simulink library "mvt_blocks"  (Simulink 3.00)
values from neighbouring files (symbols this model uses):
  stack = struct('general',[],'evaluation',[],'simulation',[],'temp',[])    [gohome.m]
libraries: mvt_blocks x1
(part 1 of 2)

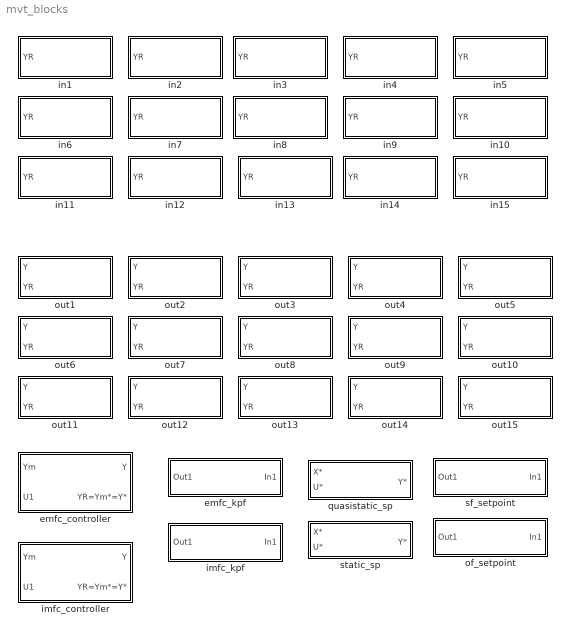
== system mvt_blocks ==
  emfc_controller : Subsystem  Orientation=left
      mask Display: disp('CONTROLLER')
  emfc_kpf : Subsystem  Orientation=left
      mask Display: disp('Kpf')
  imfc_controller : Subsystem  Orientation=left
      mask Display: disp('CONTROLLER')
  imfc_kpf : Subsystem  Orientation=left
      mask Display: disp('Kpf')
  in1 : Subsystem  Orientation=left
      mask Display: disp('COMMANDS')
  in10 : Subsystem  Orientation=left
      mask Display: disp('COMMANDS')
  in11 : Subsystem  Orientation=left
      mask Display: disp('COMMANDS')
  in12 : Subsystem  Orientation=left
      mask Display: disp('COMMANDS')
  in13 : Subsystem  Orientation=left
      mask Display: disp('COMMANDS')
  in14 : Subsystem  Orientation=left
      mask Display: disp('COMMANDS')
  in15 : Subsystem  Orientation=left
      mask Display: disp('COMMANDS')
  in2 : Subsystem  Orientation=left
      mask Display: disp('COMMANDS')
  in3 : Subsystem  Orientation=left
      mask Display: disp('COMMANDS')
  in4 : Subsystem  Orientation=left
      mask Display: disp('COMMANDS')
  in5 : Subsystem  Orientation=left
      mask Display: disp('COMMANDS')
  in6 : Subsystem  Orientation=left
      mask Display: disp('COMMANDS')
  in7 : Subsystem  Orientation=left
      mask Display: disp('COMMANDS')
  in8 : Subsystem  Orientation=left
      mask Display: disp('COMMANDS')
  in9 : Subsystem  Orientation=left
      mask Display: disp('COMMANDS')
  of_setpoint : Subsystem  Orientation=left
      mask Display: disp('Kpf')
  out1 : Subsystem
      mask Display: disp('OUTPUTS')
  out10 : Subsystem
      mask Display: disp('OUTPUTS')
  out11 : Subsystem
      mask Display: disp('OUTPUTS')
  out12 : Subsystem
      mask Display: disp('OUTPUTS')
  out13 : Subsystem
      mask Display: disp('OUTPUTS')
  out14 : Subsystem
      mask Display: disp('OUTPUTS')
  out15 : Subsystem
      mask Display: disp('OUTPUTS')
  out2 : Subsystem
      mask Display: disp('OUTPUTS')
  out3 : Subsystem
      mask Display: disp('OUTPUTS')
  out4 : Subsystem
      mask Display: disp('OUTPUTS')
  out5 : Subsystem
      mask Display: disp('OUTPUTS')
  out6 : Subsystem
      mask Display: disp('OUTPUTS')
  out7 : Subsystem
      mask Display: disp('OUTPUTS')
  out8 : Subsystem
      mask Display: disp('OUTPUTS')
  out9 : Subsystem
      mask Display: disp('OUTPUTS')
  quasistatic_sp : Subsystem  Orientation=left
      mask Display: disp('quasi-static\n SET POINT')
  sf_setpoint : Subsystem  Orientation=left
      mask Display: disp('Kpf')
  static_sp : Subsystem  Orientation=left
      mask Display: disp('static\n SET POINT')

== system mvt_blocks/emfc_controller ==
  Y : Inport  Orientation=left  Port=1  PortWidth=-1  SampleTime=-1  DataType=auto
      settings: SignalType=auto
  YR=Ym*=Y* : Inport  Orientation=left  Port=2  PortWidth=-1  SampleTime=-1  DataType=auto
      settings: SignalType=auto
  CONTROLLER : StateSpace  Orientation=left  A=stack.simulation.Ak  B=stack.simulation.Bk  C=stack.simulation.Ck  D=stack.simulation.Dk  X0=0
  MODEL : StateSpace  Orientation=left  A=stack.simulation.Am  B=stack.simulation.Bm  C=eye(size(stack.simulation.Am))  D=zeros(size(stack.simulation.Am,1),size(stack.simulation.Bm,2))  X0=0
  Matrix Gain : Subsystem  Orientation=left  mask(Matrix Gain){K=stack.simulation.Kff}
      mask prompts: K "Gain matrix:"
      mask help: Matrix Gain.
      mask Help: Multiplies input vector by entered matrix to produce output vector (y=Au).
      mask Display: disp('Kff')
  Matrix Gain1 : Subsystem  Orientation=left  mask(Matrix Gain){K=stack.simulation.Cm}
      mask prompts: K "Gain matrix:"
      mask help: Matrix Gain.
      mask Help: Multiplies input vector by entered matrix to produce output vector (y=Au).
      mask Display: disp('Cm')
  Sum : Sum  Orientation=left  Inputs=++|  SaturateOnIntegerOverflow=on
  Ym : Outport  Orientation=left  Port=1
  U1 : Outport  Orientation=left  Port=2
  wires:
  YR=Ym*=Y*/1 -> MODEL/1
  Y/1 -> CONTROLLER/1
  Matrix Gain/1(Out1) -> Sum/2
  Sum/1 -> U1/1
  CONTROLLER/1 -> Sum/1
  MODEL/1 -> Matrix Gain/1(In1), Matrix Gain1/1(In1)
  Matrix Gain1/1(Out1) -> Ym/1

== system mvt_blocks/emfc_kpf ==
  note: U*
  note: X*
  In1 : Inport  Orientation=left  Port=1  PortWidth=-1  SampleTime=-1  DataType=auto
      settings: SignalType=auto
  Matrix Gain : Subsystem  Orientation=left  mask(Matrix Gain){K=stack.simulation.Kfb}
      mask prompts: K "Gain matrix:"
      mask help: Matrix Gain.
      mask Help: Multiplies input vector by entered matrix to produce output vector (y=Au).
      mask Display: disp('Kfb')
  Matrix Gain1 : Subsystem  Orientation=left  mask(Matrix Gain){K=stack.simulation.Kpf0}
      mask prompts: K "Gain matrix:"
      mask help: Matrix Gain.
      mask Help: Multiplies input vector by entered matrix to produce output vector (y=Au).
      mask Display: disp('Kpf_0')
  Sum : Sum  Orientation=left  Inputs=++-  SaturateOnIntegerOverflow=on
  setpoint : Subsystem  Orientation=left
      mask Display: disp('SET POINT')
  Out1 : Outport  Orientation=left  Port=1
  wires:
  setpoint/1(X*) -> Matrix Gain/1(In1)
  Matrix Gain/1(Out1) -> Sum/1
  setpoint/2(U*) -> Sum/2
  Matrix Gain1/1(Out1) -> Sum/3
  In1/1 -> setpoint/1(Y*), Matrix Gain1/1(In1)
  Sum/1 -> Out1/1

== system mvt_blocks/imfc_controller ==
  Y : Inport  Orientation=left  Port=1  PortWidth=-1  SampleTime=-1  DataType=auto
      settings: SignalType=auto
  YR=Ym*=Y* : Inport  Orientation=left  Port=2  PortWidth=-1  SampleTime=-1  DataType=auto
      settings: SignalType=auto
  CONTROLLER : StateSpace  Orientation=left  A=stack.simulation.Ak  B=stack.simulation.Bk  C=stack.simulation.Ck  D=stack.simulation.Dk  X0=0
  MODEL : StateSpace  Orientation=left  A=stack.simulation.Am  B=stack.simulation.Bm  C=stack.simulation.Cm  D=stack.simulation.Dm  X0=0
  Ym : Outport  Orientation=left  Port=1
  U1 : Outport  Orientation=left  Port=2
  wires:
  Y/1 -> CONTROLLER/1
  YR=Ym*=Y*/1 -> MODEL/1
  MODEL/1 -> Ym/1
  CONTROLLER/1 -> U1/1

== system mvt_blocks/imfc_kpf ==
  note: X*
  note: U*
  In1 : Inport  Orientation=left  Port=1  PortWidth=-1  SampleTime=-1  DataType=auto
      settings: SignalType=auto
  Matrix Gain : Subsystem  Orientation=left  mask(Matrix Gain){K=stack.simulation.Kfb}
      mask prompts: K "Gain matrix:"
      mask help: Matrix Gain.
      mask Help: Multiplies input vector by entered matrix to produce output vector (y=Au).
      mask Display: disp('Kfb')
  Sum : Sum  Orientation=left  Inputs=|++  SaturateOnIntegerOverflow=on
  setpoint : Subsystem  Orientation=left
      mask Display: disp('SET POINT')
  Out1 : Outport  Orientation=left  Port=1
  wires:
  Sum/1 -> Out1/1
  setpoint/2(U*) -> Sum/2
  Matrix Gain/1(Out1) -> Sum/1
  setpoint/1(X*) -> Matrix Gain/1(In1)
  In1/1 -> setpoint/1(Y*)

== system mvt_blocks/in1 ==
  note: YR1
  Gen 1 : SignalGenerator  Orientation=left  WaveForm=sine  Amplitude=0.000000  Frequency=1  Units=rad/sec
  Step 1 : Step  Orientation=left  Time=0  Before=0  After=1  SampleTime=0
  Sum : Sum  Orientation=left  Inputs=|++  SaturateOnIntegerOverflow=on
  YR : Outport  Orientation=left  Port=1
  wires:
  Step 1/1 -> Sum/2
  Gen 1/1 -> Sum/1
  Sum/1 -> YR/1

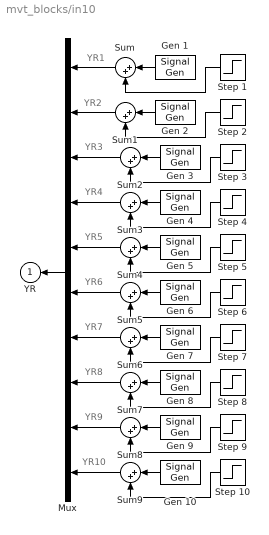
== system mvt_blocks/in10 ==
  note: YR1
  note: YR2
  note: YR3
  note: YR4
  note: YR5
  note: YR6
  note: YR7
  note: YR8
  note: YR9
  note: YR10
  Gen {1..10} (10 alike) : SignalGenerator  Orientation=left  WaveForm=sine  Amplitude=0.000000  Frequency=1  Units=rad/sec
  Mux : Mux  Orientation=left  Inputs=10
  Step {1..10} (10 alike) : Step  Orientation=left  Time=0  Before=0  After=1  SampleTime=0
  Sum{,1..9} (10 alike) : Sum  Orientation=left  Inputs=|++  SaturateOnIntegerOverflow=on
  YR : Outport  Orientation=left  Port=1
  wires:
  Sum/1 -> Mux/1
  Sum1/1 -> Mux/2
  Gen 1/1 -> Sum/1
  Mux/1 -> YR/1
  Sum3/1 -> Mux/4
  Sum4/1 -> Mux/5
  Step 1/1 -> Sum/2
  Gen 2/1 -> Sum1/1
  Step 2/1 -> Sum1/2
  Sum2/1 -> Mux/3
  Gen 3/1 -> Sum2/1
  Step 3/1 -> Sum2/2
  Gen 4/1 -> Sum3/1
  Step 4/1 -> Sum3/2
  Gen 5/1 -> Sum4/1
  Step 5/1 -> Sum4/2
  Sum5/1 -> Mux/6
  Gen 6/1 -> Sum5/1
  Step 6/1 -> Sum5/2
  Sum6/1 -> Mux/7
  Gen 7/1 -> Sum6/1
  Step 7/1 -> Sum6/2
  Sum7/1 -> Mux/8
  Gen 8/1 -> Sum7/1
  Step 8/1 -> Sum7/2
  Sum8/1 -> Mux/9
  Gen 9/1 -> Sum8/1
  Step 9/1 -> Sum8/2
  Sum9/1 -> Mux/10
  Gen 10/1 -> Sum9/1
  Step 10/1 -> Sum9/2

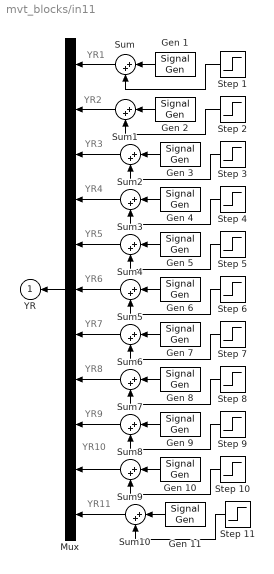
== system mvt_blocks/in11 ==
  note: YR1
  note: YR2
  note: YR3
  note: YR4
  note: YR5
  note: YR6
  note: YR7
  note: YR8
  note: YR9
  note: YR10
  note: YR11
  Gen {1..11} (11 alike) : SignalGenerator  Orientation=left  WaveForm=sine  Amplitude=0.000000  Frequency=1  Units=rad/sec
  Mux : Mux  Orientation=left  Inputs=11
  Step {1..11} (11 alike) : Step  Orientation=left  Time=0  Before=0  After=1  SampleTime=0
  Sum{,1..10} (11 alike) : Sum  Orientation=left  Inputs=|++  SaturateOnIntegerOverflow=on
  YR : Outport  Orientation=left  Port=1
  wires:
  Sum/1 -> Mux/1
  Sum1/1 -> Mux/2
  Gen 1/1 -> Sum/1
  Mux/1 -> YR/1
  Sum3/1 -> Mux/4
  Sum4/1 -> Mux/5
  Gen 2/1 -> Sum1/1
  Sum2/1 -> Mux/3
  Gen 3/1 -> Sum2/1
  Step 3/1 -> Sum2/2
  Gen 4/1 -> Sum3/1
  Step 4/1 -> Sum3/2
  Gen 5/1 -> Sum4/1
  Step 5/1 -> Sum4/2
  Sum5/1 -> Mux/6
  Gen 6/1 -> Sum5/1
  Step 6/1 -> Sum5/2
  Sum6/1 -> Mux/7
  Gen 7/1 -> Sum6/1
  Step 7/1 -> Sum6/2
  Sum7/1 -> Mux/8
  Gen 8/1 -> Sum7/1
  Step 8/1 -> Sum7/2
  Sum8/1 -> Mux/9
  Gen 9/1 -> Sum8/1
  Step 9/1 -> Sum8/2
  Sum9/1 -> Mux/10
  Gen 10/1 -> Sum9/1
  Step 10/1 -> Sum9/2
  Step 1/1 -> Sum/2
  Step 2/1 -> Sum1/2
  Sum10/1 -> Mux/11
  Gen 11/1 -> Sum10/1
  Step 11/1 -> Sum10/2

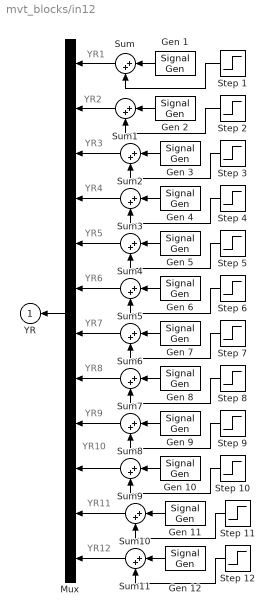
== system mvt_blocks/in12 ==
  note: YR1
  note: YR2
  note: YR3
  note: YR4
  note: YR5
  note: YR6
  note: YR7
  note: YR8
  note: YR9
  note: YR10
  note: YR11
  note: YR12
  Gen {1..12} (12 alike) : SignalGenerator  Orientation=left  WaveForm=sine  Amplitude=0.000000  Frequency=1  Units=rad/sec
  Mux : Mux  Orientation=left  Inputs=12
  Step {1..12} (12 alike) : Step  Orientation=left  Time=0  Before=0  After=1  SampleTime=0
  Sum{,1..11} (12 alike) : Sum  Orientation=left  Inputs=|++  SaturateOnIntegerOverflow=on
  YR : Outport  Orientation=left  Port=1
  wires:
  Sum/1 -> Mux/1
  Sum1/1 -> Mux/2
  Gen 1/1 -> Sum/1
  Mux/1 -> YR/1
  Sum3/1 -> Mux/4
  Sum4/1 -> Mux/5
  Gen 2/1 -> Sum1/1
  Sum2/1 -> Mux/3
  Gen 3/1 -> Sum2/1
  Step 3/1 -> Sum2/2
  Gen 4/1 -> Sum3/1
  Step 4/1 -> Sum3/2
  Gen 5/1 -> Sum4/1
  Step 5/1 -> Sum4/2
  Sum5/1 -> Mux/6
  Gen 6/1 -> Sum5/1
  Step 6/1 -> Sum5/2
  Sum6/1 -> Mux/7
  Gen 7/1 -> Sum6/1
  Step 7/1 -> Sum6/2
  Sum7/1 -> Mux/8
  Gen 8/1 -> Sum7/1
  Step 8/1 -> Sum7/2
  Sum8/1 -> Mux/9
  Gen 9/1 -> Sum8/1
  Step 9/1 -> Sum8/2
  Sum9/1 -> Mux/10
  Gen 10/1 -> Sum9/1
  Step 10/1 -> Sum9/2
  Step 1/1 -> Sum/2
  Step 2/1 -> Sum1/2
  Sum10/1 -> Mux/11
  Gen 11/1 -> Sum10/1
  Step 11/1 -> Sum10/2
  Sum11/1 -> Mux/12
  Gen 12/1 -> Sum11/1
  Step 12/1 -> Sum11/2

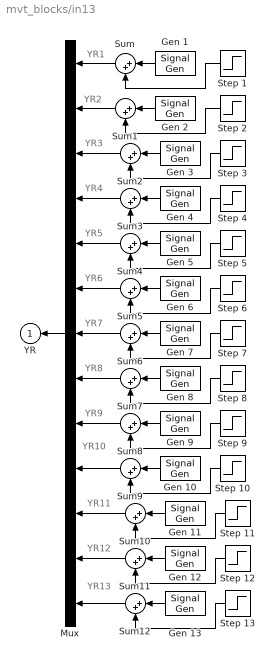
== system mvt_blocks/in13 ==
  note: YR1
  note: YR2
  note: YR3
  note: YR4
  note: YR5
  note: YR6
  note: YR7
  note: YR8
  note: YR9
  note: YR10
  note: YR11
  note: YR12
  note: YR13
  Gen {1..10,13} (11 alike) : SignalGenerator  Orientation=left  WaveForm=sine  Amplitude=0.000000  Frequency=1  Units=rad/sec
  Gen 11 : SignalGenerator  Orientation=left  WaveForm=sine  Amplitude=0.000000  Frequency=0.000000  Units=rad/sec
  Gen 12 : SignalGenerator  Orientation=left  WaveForm=sine  Amplitude=0.000000  Frequency=0.000000  Units=rad/sec
  Mux : Mux  Orientation=left  Inputs=13
  Step {1..13} (13 alike) : Step  Orientation=left  Time=0  Before=0  After=1  SampleTime=0
  Sum{,1..12} (13 alike) : Sum  Orientation=left  Inputs=|++  SaturateOnIntegerOverflow=on
  YR : Outport  Orientation=left  Port=1
  wires:
  Sum/1 -> Mux/1
  Sum1/1 -> Mux/2
  Gen 1/1 -> Sum/1
  Mux/1 -> YR/1
  Sum3/1 -> Mux/4
  Sum4/1 -> Mux/5
  Gen 2/1 -> Sum1/1
  Sum2/1 -> Mux/3
  Gen 3/1 -> Sum2/1
  Step 3/1 -> Sum2/2
  Gen 4/1 -> Sum3/1
  Step 4/1 -> Sum3/2
  Gen 5/1 -> Sum4/1
  Step 5/1 -> Sum4/2
  Sum5/1 -> Mux/6
  Gen 6/1 -> Sum5/1
  Step 6/1 -> Sum5/2
  Sum6/1 -> Mux/7
  Gen 7/1 -> Sum6/1
  Step 7/1 -> Sum6/2
  Sum7/1 -> Mux/8
  Gen 8/1 -> Sum7/1
  Step 8/1 -> Sum7/2
  Sum8/1 -> Mux/9
  Gen 9/1 -> Sum8/1
  Step 9/1 -> Sum8/2
  Sum9/1 -> Mux/10
  Gen 10/1 -> Sum9/1
  Step 10/1 -> Sum9/2
  Sum10/1 -> Mux/11
  Gen 11/1 -> Sum10/1
  Step 11/1 -> Sum10/2
  Sum11/1 -> Mux/12
  Gen 12/1 -> Sum11/1
  Step 12/1 -> Sum11/2
  Sum12/1 -> Mux/13
  Gen 13/1 -> Sum12/1
  Step 1/1 -> Sum/2
  Step 2/1 -> Sum1/2
  Step 13/1 -> Sum12/2

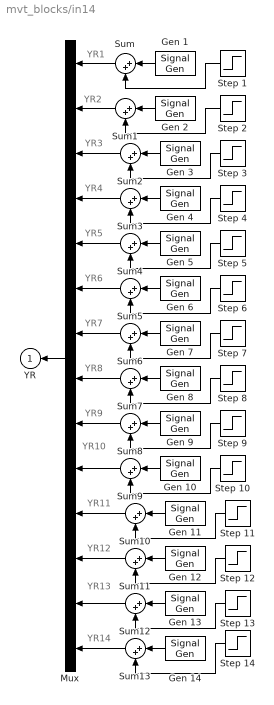
== system mvt_blocks/in14 ==
  note: YR14
  note: YR1
  note: YR2
  note: YR3
  note: YR4
  note: YR5
  note: YR6
  note: YR7
  note: YR8
  note: YR9
  note: YR10
  note: YR11
  note: YR12
  note: YR13
  Gen {1..14} (14 alike) : SignalGenerator  Orientation=left  WaveForm=sine  Amplitude=0.000000  Frequency=1  Units=rad/sec
  Mux : Mux  Orientation=left  Inputs=14
  Step {1..14} (14 alike) : Step  Orientation=left  Time=0  Before=0  After=1  SampleTime=0
  Sum{,1..13} (14 alike) : Sum  Orientation=left  Inputs=|++  SaturateOnIntegerOverflow=on
  YR : Outport  Orientation=left  Port=1
  wires:
  Step 2/1 -> Sum1/2
  Step 1/1 -> Sum/2
  Step 13/1 -> Sum12/2
  Gen 13/1 -> Sum12/1
  Sum12/1 -> Mux/13
  Step 12/1 -> Sum11/2
  Gen 12/1 -> Sum11/1
  Sum11/1 -> Mux/12
  Step 11/1 -> Sum10/2
  Gen 11/1 -> Sum10/1
  Sum10/1 -> Mux/11
  Step 10/1 -> Sum9/2
  Gen 10/1 -> Sum9/1
  Sum9/1 -> Mux/10
  Step 9/1 -> Sum8/2
  Gen 9/1 -> Sum8/1
  Sum8/1 -> Mux/9
  Step 8/1 -> Sum7/2
  Gen 8/1 -> Sum7/1
  Sum7/1 -> Mux/8
  Step 7/1 -> Sum6/2
  Gen 7/1 -> Sum6/1
  Sum6/1 -> Mux/7
  Step 6/1 -> Sum5/2
  Gen 6/1 -> Sum5/1
  Sum5/1 -> Mux/6
  Step 5/1 -> Sum4/2
  Gen 5/1 -> Sum4/1
  Step 4/1 -> Sum3/2
  Gen 4/1 -> Sum3/1
  Step 3/1 -> Sum2/2
  Gen 3/1 -> Sum2/1
  Sum2/1 -> Mux/3
  Gen 2/1 -> Sum1/1
  Sum4/1 -> Mux/5
  Sum3/1 -> Mux/4
  Mux/1 -> YR/1
  Gen 1/1 -> Sum/1
  Sum1/1 -> Mux/2
  Sum/1 -> Mux/1
  Gen 14/1 -> Sum13/1
  Sum13/1 -> Mux/14
  Step 14/1 -> Sum13/2

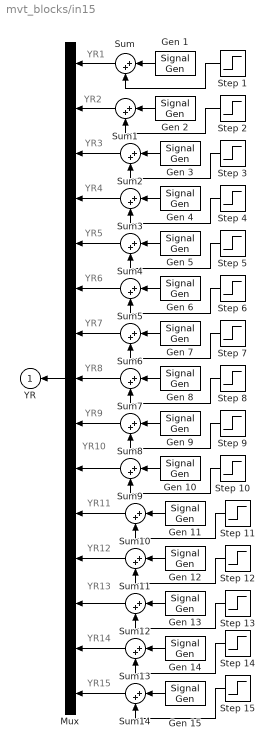
== system mvt_blocks/in15 ==
  note: YR14
  note: YR1
  note: YR2
  note: YR3
  note: YR4
  note: YR5
  note: YR6
  note: YR7
  note: YR8
  note: YR9
  note: YR10
  note: YR11
  note: YR12
  note: YR13
  note: YR15
  Gen {1..15} (15 alike) : SignalGenerator  Orientation=left  WaveForm=sine  Amplitude=0.000000  Frequency=1  Units=rad/sec
  Mux : Mux  Orientation=left  Inputs=15
  Step {1..15} (15 alike) : Step  Orientation=left  Time=0  Before=0  After=1  SampleTime=0
  Sum{,1..14} (15 alike) : Sum  Orientation=left  Inputs=|++  SaturateOnIntegerOverflow=on
  YR : Outport  Orientation=left  Port=1
  wires:
  Step 14/1 -> Sum13/2
  Sum13/1 -> Mux/14
  Gen 14/1 -> Sum13/1
  Sum/1 -> Mux/1
  Sum1/1 -> Mux/2
  Gen 1/1 -> Sum/1
  Mux/1 -> YR/1
  Sum3/1 -> Mux/4
  Sum4/1 -> Mux/5
  Gen 2/1 -> Sum1/1
  Sum2/1 -> Mux/3
  Gen 3/1 -> Sum2/1
  Step 3/1 -> Sum2/2
  Gen 4/1 -> Sum3/1
  Step 4/1 -> Sum3/2
  Gen 5/1 -> Sum4/1
  Step 5/1 -> Sum4/2
  Sum5/1 -> Mux/6
  Gen 6/1 -> Sum5/1
  Step 6/1 -> Sum5/2
  Sum6/1 -> Mux/7
  Gen 7/1 -> Sum6/1
  Step 7/1 -> Sum6/2
  Sum7/1 -> Mux/8
  Gen 8/1 -> Sum7/1
  Step 8/1 -> Sum7/2
  Sum8/1 -> Mux/9
  Gen 9/1 -> Sum8/1
  Step 9/1 -> Sum8/2
  Sum9/1 -> Mux/10
  Gen 10/1 -> Sum9/1
  Step 10/1 -> Sum9/2
  Sum10/1 -> Mux/11
  Gen 11/1 -> Sum10/1
  Step 11/1 -> Sum10/2
  Sum11/1 -> Mux/12
  Gen 12/1 -> Sum11/1
  Step 12/1 -> Sum11/2
  Sum12/1 -> Mux/13
  Gen 13/1 -> Sum12/1
  Step 13/1 -> Sum12/2
  Step 1/1 -> Sum/2
  Step 2/1 -> Sum1/2
  Step 15/1 -> Sum14/2
  Sum14/1 -> Mux/15
  Gen 15/1 -> Sum14/1

== system mvt_blocks/in2 ==
  note: YR2
  note: YR1
  Gen 1 : SignalGenerator  Orientation=left  WaveForm=sine  Amplitude=0.000000  Frequency=1  Units=rad/sec
  Gen 2 : SignalGenerator  Orientation=left  WaveForm=sine  Amplitude=0.000000  Frequency=1  Units=rad/sec
  Mux : Mux  Orientation=left  Inputs=2
  Step 1 : Step  Orientation=left  Time=0  Before=0  After=1  SampleTime=0
  Step 2 : Step  Orientation=left  Time=0  Before=0  After=1  SampleTime=0
  Sum : Sum  Orientation=left  Inputs=|++  SaturateOnIntegerOverflow=on
  Sum1 : Sum  Orientation=left  Inputs=|++  SaturateOnIntegerOverflow=on
  YR : Outport  Orientation=left  Port=1
  wires:
  Mux/1 -> YR/1
  Gen 1/1 -> Sum/1
  Step 2/1 -> Sum1/2
  Gen 2/1 -> Sum1/1
  Sum1/1 -> Mux/2
  Step 1/1 -> Sum/2
  Sum/1 -> Mux/1

== system mvt_blocks/in3 ==
  note: YR1
  note: YR2
  note: YR3
  Gen 1 : SignalGenerator  Orientation=left  WaveForm=sine  Amplitude=0.000000  Frequency=1  Units=rad/sec
  Gen 2 : SignalGenerator  Orientation=left  WaveForm=sine  Amplitude=0.000000  Frequency=1  Units=rad/sec
  Gen 3 : SignalGenerator  Orientation=left  WaveForm=sine  Amplitude=0.000000  Frequency=1  Units=rad/sec
  Mux : Mux  Orientation=left  Inputs=3
  Step 1 : Step  Orientation=left  Time=0  Before=0  After=1  SampleTime=0
  Step 2 : Step  Orientation=left  Time=0  Before=0  After=1  SampleTime=0
  Step 3 : Step  Orientation=left  Time=0  Before=0  After=1  SampleTime=0
  Sum : Sum  Orientation=left  Inputs=|++  SaturateOnIntegerOverflow=on
  Sum1 : Sum  Orientation=left  Inputs=|++  SaturateOnIntegerOverflow=on
  Sum2 : Sum  Orientation=left  Inputs=|++  SaturateOnIntegerOverflow=on
  YR : Outport  Orientation=left  Port=1
  wires:
  Sum/1 -> Mux/1
  Step 1/1 -> Sum/2
  Sum1/1 -> Mux/2
  Gen 2/1 -> Sum1/1
  Step 2/1 -> Sum1/2
  Gen 1/1 -> Sum/1
  Mux/1 -> YR/1
  Gen 3/1 -> Sum2/1
  Step 3/1 -> Sum2/2
  Sum2/1 -> Mux/3

== system mvt_blocks/in4 ==
  note: YR4
  note: YR3
  note: YR2
  note: YR1
  Gen {1..4} (4 alike) : SignalGenerator  Orientation=left  WaveForm=sine  Amplitude=0.000000  Frequency=1  Units=rad/sec
  Mux : Mux  Orientation=left  Inputs=4
  Step {1..4} (4 alike) : Step  Orientation=left  Time=0  Before=0  After=1  SampleTime=0
  Sum{,1..3} (4 alike) : Sum  Orientation=left  Inputs=|++  SaturateOnIntegerOverflow=on
  YR : Outport  Orientation=left  Port=1
  wires:
  Sum3/1 -> Mux/4
  Step 4/1 -> Sum3/2
  Gen 4/1 -> Sum3/1
  Sum2/1 -> Mux/3
  Step 3/1 -> Sum2/2
  Gen 3/1 -> Sum2/1
  Mux/1 -> YR/1
  Gen 1/1 -> Sum/1
  Step 2/1 -> Sum1/2
  Gen 2/1 -> Sum1/1
  Sum1/1 -> Mux/2
  Step 1/1 -> Sum/2
  Sum/1 -> Mux/1

== system mvt_blocks/in5 ==
  note: YR1
  note: YR2
  note: YR3
  note: YR4
  note: YR5
  Gen {1..5} (5 alike) : SignalGenerator  Orientation=left  WaveForm=sine  Amplitude=0.000000  Frequency=1  Units=rad/sec
  Mux : Mux  Orientation=left  Inputs=5
  Step {1..5} (5 alike) : Step  Orientation=left  Time=0  Before=0  After=1  SampleTime=0
  Sum{,1..4} (5 alike) : Sum  Orientation=left  Inputs=|++  SaturateOnIntegerOverflow=on
  YR : Outport  Orientation=left  Port=1
  wires:
  Sum/1 -> Mux/1
  Step 1/1 -> Sum/2
  Sum1/1 -> Mux/2
  Gen 2/1 -> Sum1/1
  Step 2/1 -> Sum1/2
  Gen 1/1 -> Sum/1
  Mux/1 -> YR/1
  Gen 3/1 -> Sum2/1
  Step 3/1 -> Sum2/2
  Sum2/1 -> Mux/3
  Gen 4/1 -> Sum3/1
  Step 4/1 -> Sum3/2
  Sum3/1 -> Mux/4
  Gen 5/1 -> Sum4/1
  Step 5/1 -> Sum4/2
  Sum4/1 -> Mux/5

== system mvt_blocks/in6 ==
  note: YR1
  note: YR2
  note: YR3
  note: YR4
  note: YR5
  note: YR6
  Gen {1..6} (6 alike) : SignalGenerator  Orientation=left  WaveForm=sine  Amplitude=0.000000  Frequency=1  Units=rad/sec
  Mux : Mux  Orientation=left  Inputs=6
  Step {1..6} (6 alike) : Step  Orientation=left  Time=0  Before=0  After=1  SampleTime=0
  Sum{,1..5} (6 alike) : Sum  Orientation=left  Inputs=|++  SaturateOnIntegerOverflow=on
  YR : Outport  Orientation=left  Port=1
  wires:
  Sum/1 -> Mux/1
  Step 1/1 -> Sum/2
  Sum1/1 -> Mux/2
  Gen 2/1 -> Sum1/1
  Step 2/1 -> Sum1/2
  Gen 1/1 -> Sum/1
  Mux/1 -> YR/1
  Gen 3/1 -> Sum2/1
  Step 3/1 -> Sum2/2
  Sum2/1 -> Mux/3
  Gen 4/1 -> Sum3/1
  Step 4/1 -> Sum3/2
  Sum3/1 -> Mux/4
  Gen 5/1 -> Sum4/1
  Step 5/1 -> Sum4/2
  Sum4/1 -> Mux/5
  Gen 6/1 -> Sum5/1
  Step 6/1 -> Sum5/2
  Sum5/1 -> Mux/6

== system mvt_blocks/in7 ==
  note: YR1
  note: YR2
  note: YR3
  note: YR4
  note: YR5
  note: YR6
  note: YR7
  Gen {1..7} (7 alike) : SignalGenerator  Orientation=left  WaveForm=sine  Amplitude=0.000000  Frequency=1  Units=rad/sec
  Mux : Mux  Orientation=left  Inputs=7
  Step {1..7} (7 alike) : Step  Orientation=left  Time=0  Before=0  After=1  SampleTime=0
  Sum{,1..6} (7 alike) : Sum  Orientation=left  Inputs=|++  SaturateOnIntegerOverflow=on
  YR : Outport  Orientation=left  Port=1
  wires:
  Sum/1 -> Mux/1
  Step 1/1 -> Sum/2
  Sum1/1 -> Mux/2
  Gen 2/1 -> Sum1/1
  Step 2/1 -> Sum1/2
  Gen 1/1 -> Sum/1
  Mux/1 -> YR/1
  Gen 3/1 -> Sum2/1
  Step 3/1 -> Sum2/2
  Sum2/1 -> Mux/3
  Gen 4/1 -> Sum3/1
  Step 4/1 -> Sum3/2
  Sum3/1 -> Mux/4
  Gen 5/1 -> Sum4/1
  Step 5/1 -> Sum4/2
  Sum4/1 -> Mux/5
  Gen 6/1 -> Sum5/1
  Step 6/1 -> Sum5/2
  Sum5/1 -> Mux/6
  Gen 7/1 -> Sum6/1
  Step 7/1 -> Sum6/2
  Sum6/1 -> Mux/7

== system mvt_blocks/in8 ==
  note: YR8
  note: YR7
  note: YR6
  note: YR5
  note: YR4
  note: YR3
  note: YR2
  note: YR1
  Gen {1..8} (8 alike) : SignalGenerator  Orientation=left  WaveForm=sine  Amplitude=0.000000  Frequency=1  Units=rad/sec
  Mux : Mux  Orientation=left  Inputs=8
  Step {1..8} (8 alike) : Step  Orientation=left  Time=0  Before=0  After=1  SampleTime=0
  Sum{,1..7} (8 alike) : Sum  Orientation=left  Inputs=|++  SaturateOnIntegerOverflow=on
  YR : Outport  Orientation=left  Port=1
  wires:
  Sum/1 -> Mux/1
  Sum1/1 -> Mux/2
  Gen 1/1 -> Sum/1
  Mux/1 -> YR/1
  Sum3/1 -> Mux/4
  Sum4/1 -> Mux/5
  Step 1/1 -> Sum/2
  Gen 2/1 -> Sum1/1
  Step 2/1 -> Sum1/2
  Sum2/1 -> Mux/3
  Gen 3/1 -> Sum2/1
  Step 3/1 -> Sum2/2
  Gen 4/1 -> Sum3/1
  Step 4/1 -> Sum3/2
  Gen 5/1 -> Sum4/1
  Step 5/1 -> Sum4/2
  Sum5/1 -> Mux/6
  Gen 6/1 -> Sum5/1
  Step 6/1 -> Sum5/2
  Sum6/1 -> Mux/7
  Gen 7/1 -> Sum6/1
  Step 7/1 -> Sum6/2
  Sum7/1 -> Mux/8
  Gen 8/1 -> Sum7/1
  Step 8/1 -> Sum7/2

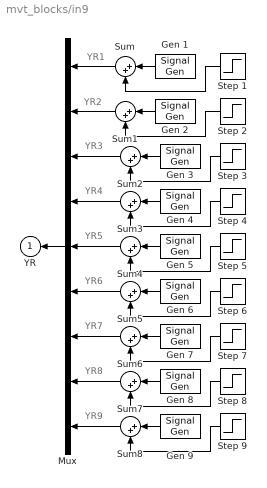
== system mvt_blocks/in9 ==
  note: YR1
  note: YR2
  note: YR3
  note: YR4
  note: YR5
  note: YR6
  note: YR7
  note: YR8
  note: YR9
  Gen {1..9} (9 alike) : SignalGenerator  Orientation=left  WaveForm=sine  Amplitude=0.000000  Frequency=1  Units=rad/sec
  Mux : Mux  Orientation=left  Inputs=9
  Step {1..9} (9 alike) : Step  Orientation=left  Time=0  Before=0  After=1  SampleTime=0
  Sum{,1..8} (9 alike) : Sum  Orientation=left  Inputs=|++  SaturateOnIntegerOverflow=on
  YR : Outport  Orientation=left  Port=1
  wires:
  Sum/1 -> Mux/1
  Sum1/1 -> Mux/2
  Gen 1/1 -> Sum/1
  Mux/1 -> YR/1
  Sum3/1 -> Mux/4
  Sum4/1 -> Mux/5
  Step 1/1 -> Sum/2
  Gen 2/1 -> Sum1/1
  Step 2/1 -> Sum1/2
  Sum2/1 -> Mux/3
  Gen 3/1 -> Sum2/1
  Step 3/1 -> Sum2/2
  Gen 4/1 -> Sum3/1
  Step 4/1 -> Sum3/2
  Gen 5/1 -> Sum4/1
  Step 5/1 -> Sum4/2
  Sum5/1 -> Mux/6
  Gen 6/1 -> Sum5/1
  Step 6/1 -> Sum5/2
  Sum6/1 -> Mux/7
  Gen 7/1 -> Sum6/1
  Step 7/1 -> Sum6/2
  Sum7/1 -> Mux/8
  Gen 8/1 -> Sum7/1
  Step 8/1 -> Sum7/2
  Sum8/1 -> Mux/9
  Gen 9/1 -> Sum8/1
  Step 9/1 -> Sum8/2

== system mvt_blocks/of_setpoint ==
  note: X*
  note: U*
  In1 : Inport  Orientation=left  Port=1  PortWidth=-1  SampleTime=-1  DataType=auto
      settings: SignalType=auto
  SubSystem : Subsystem  Orientation=left
      mask Display: disp('Kfb')
  Sum : Sum  Orientation=left  Inputs=|++  SaturateOnIntegerOverflow=on
  setpoint : mvt_blocks/sf_setpoint/setpoint  Orientation=left
  Out1 : Outport  Orientation=left  Port=1
  wires:
  Sum/1 -> Out1/1
  SubSystem/1(Kof Y*) -> Sum/1
  setpoint/1 -> SubSystem/1(X*)
  In1/1 -> setpoint/1
  setpoint/2 -> Sum/2, SubSystem/2(U*)

== system mvt_blocks/out1 ==
  Y : Inport  Port=1  PortWidth=-1  SampleTime=0  DataType=auto
      settings: SignalType=auto
  YR : Inport  Port=2  PortWidth=-1  SampleTime=0  DataType=auto
      settings: SignalType=auto
  " 1" : Scope
      settings: Orientation=up  TimeRange=100.000000  YMin=-2  YMax=2  SaveToWorkspace=off  SaveName=ScopeData  DataFormat=Matrix
  Mux : Mux  Orientation=up  Inputs=2
  wires:
  Mux/1 -> " 1"/1
  Y/1 -> Mux/1
  YR/1 -> Mux/2

== system mvt_blocks/out10 ==
  Y : Inport  Port=1  PortWidth=-1  SampleTime=0  DataType=auto
      settings: SignalType=auto
  YR : Inport  Port=2  PortWidth=-1  SampleTime=0  DataType=auto
      settings: SignalType=auto
   {1..10} (10 alike) : Scope
      " 1" settings: Orientation=up  TimeRange=100.000000  YMin=-2  YMax=2  SaveToWorkspace=off  SaveName=ScopeData  DataFormat=Matrix
      " 10" settings: Orientation=up  TimeRange=100.000000  YMin=-2.000000  YMax=2.000000  SaveToWorkspace=off  SaveName=ScopeData  DataFormat=Matrix
      " 2" settings: Orientation=up  TimeRange=100.000000  YMin=-2.000000  YMax=2.000000  SaveToWorkspace=off  SaveName=ScopeData  DataFormat=Matrix
      " 3" settings: Orientation=up  TimeRange=100.000000  YMin=-2.000000  YMax=2.000000  SaveToWorkspace=off  SaveName=ScopeData  DataFormat=Matrix
      " 4" settings: Orientation=up  TimeRange=100.000000  YMin=-2.000000  YMax=2.000000  SaveToWorkspace=off  SaveName=ScopeData  DataFormat=Matrix
      " 5" settings: Orientation=up  TimeRange=100.000000  YMin=-2.000000  YMax=2.000000  SaveToWorkspace=off  SaveName=ScopeData  DataFormat=Matrix
      " 6" settings: Orientation=up  TimeRange=100.000000  YMin=-2.000000  YMax=2.000000  SaveToWorkspace=off  SaveName=ScopeData  DataFormat=Matrix
      " 7" settings: Orientation=up  TimeRange=100.000000  YMin=-2.000000  YMax=2.000000  SaveToWorkspace=off  SaveName=ScopeData  DataFormat=Matrix
      " 8" settings: Orientation=up  TimeRange=100.000000  YMin=-2.000000  YMax=2.000000  SaveToWorkspace=off  SaveName=ScopeData  DataFormat=Matrix
      " 9" settings: Orientation=up  TimeRange=100.000000  YMin=-2.000000  YMax=2.000000  SaveToWorkspace=off  SaveName=ScopeData  DataFormat=Matrix
  Demux : Demux  Outputs=10
  Demux1 : Demux  Outputs=10
  Mux{,1..9} (10 alike) : Mux  Orientation=up  Inputs=2
  wires:
  Y/1 -> Demux/1
  Mux/1 -> " 1"/1
  Demux/3 -> Mux2/1
  Demux/1 -> Mux/1
  YR/1 -> Demux1/1
  Demux1/2 -> Mux1/2
  Demux1/3 -> Mux2/2
  Demux/4 -> Mux3/1
  Demux/2 -> Mux1/1
  Demux/5 -> Mux4/1
  Demux1/5 -> Mux4/2
  Demux/6 -> Mux5/1
  Demux1/6 -> Mux5/2
  Demux/7 -> Mux6/1
  Demux1/7 -> Mux6/2
  Mux1/1 -> " 2"/1
  Mux2/1 -> " 3"/1
  Mux3/1 -> " 4"/1
  Mux4/1 -> " 5"/1
  Mux5/1 -> " 6"/1
  Mux6/1 -> " 7"/1
  Mux7/1 -> " 8"/1
  Demux/8 -> Mux7/1
  Demux1/8 -> Mux7/2
  Demux1/1 -> Mux/2
  Mux8/1 -> " 9"/1
  Demux/9 -> Mux8/1
  Demux1/9 -> Mux8/2
  Demux1/4 -> Mux3/2
  Mux9/1 -> " 10"/1
  Demux/10 -> Mux9/1
  Demux1/10 -> Mux9/2

== system mvt_blocks/out11 ==
  Y : Inport  Port=1  PortWidth=-1  SampleTime=0  DataType=auto
      settings: SignalType=auto
  YR : Inport  Port=2  PortWidth=-1  SampleTime=0  DataType=auto
      settings: SignalType=auto
   {1..11} (11 alike) : Scope
      " 1" settings: Orientation=up  TimeRange=100.000000  YMin=-2  YMax=2  SaveToWorkspace=off  SaveName=ScopeData  DataFormat=Matrix
      " 10" settings: Orientation=up  TimeRange=100.000000  YMin=-2.000000  YMax=2.000000  SaveToWorkspace=off  SaveName=ScopeData  DataFormat=Matrix
      " 11" settings: Orientation=up  TimeRange=100.000000  YMin=-2.000000  YMax=2.000000  SaveToWorkspace=off  SaveName=ScopeData  DataFormat=Matrix
      " 2" settings: Orientation=up  TimeRange=100.000000  YMin=-2.000000  YMax=2.000000  SaveToWorkspace=off  SaveName=ScopeData  DataFormat=Matrix
      " 3" settings: Orientation=up  TimeRange=100.000000  YMin=-2.000000  YMax=2.000000  SaveToWorkspace=off  SaveName=ScopeData  DataFormat=Matrix
      " 4" settings: Orientation=up  TimeRange=100.000000  YMin=-2.000000  YMax=2.000000  SaveToWorkspace=off  SaveName=ScopeData  DataFormat=Matrix
      " 5" settings: Orientation=up  TimeRange=100.000000  YMin=-2.000000  YMax=2.000000  SaveToWorkspace=off  SaveName=ScopeData  DataFormat=Matrix
      " 6" settings: Orientation=up  TimeRange=100.000000  YMin=-2.000000  YMax=2.000000  SaveToWorkspace=off  SaveName=ScopeData  DataFormat=Matrix
      " 7" settings: Orientation=up  TimeRange=100.000000  YMin=-2.000000  YMax=2.000000  SaveToWorkspace=off  SaveName=ScopeData  DataFormat=Matrix
      " 8" settings: Orientation=up  TimeRange=100.000000  YMin=-2.000000  YMax=2.000000  SaveToWorkspace=off  SaveName=ScopeData  DataFormat=Matrix
      " 9" settings: Orientation=up  TimeRange=100.000000  YMin=-2.000000  YMax=2.000000  SaveToWorkspace=off  SaveName=ScopeData  DataFormat=Matrix
  Demux : Demux  Outputs=11
  Demux1 : Demux  Outputs=11
  Mux{,1..10} (11 alike) : Mux  Orientation=up  Inputs=2
  wires:
  Y/1 -> Demux/1
  Mux/1 -> " 1"/1
  Demux/3 -> Mux2/1
  Demux/1 -> Mux/1
  YR/1 -> Demux1/1
  Demux1/2 -> Mux1/2
  Demux1/3 -> Mux2/2
  Demux/4 -> Mux3/1
  Demux/2 -> Mux1/1
  Demux/5 -> Mux4/1
  Demux1/5 -> Mux4/2
  Demux/6 -> Mux5/1
  Demux1/6 -> Mux5/2
  Demux/7 -> Mux6/1
  Demux1/7 -> Mux6/2
  Mux1/1 -> " 2"/1
  Mux2/1 -> " 3"/1
  Mux3/1 -> " 4"/1
  Mux4/1 -> " 5"/1
  Mux5/1 -> " 6"/1
  Mux6/1 -> " 7"/1
  Mux7/1 -> " 8"/1
  Demux/8 -> Mux7/1
  Demux1/8 -> Mux7/2
  Demux1/1 -> Mux/2
  Mux8/1 -> " 9"/1
  Demux/9 -> Mux8/1
  Demux1/9 -> Mux8/2
  Demux1/4 -> Mux3/2
  Mux9/1 -> " 10"/1
  Demux/10 -> Mux9/1
  Demux1/10 -> Mux9/2
  Mux10/1 -> " 11"/1
  Demux/11 -> Mux10/1
  Demux1/11 -> Mux10/2

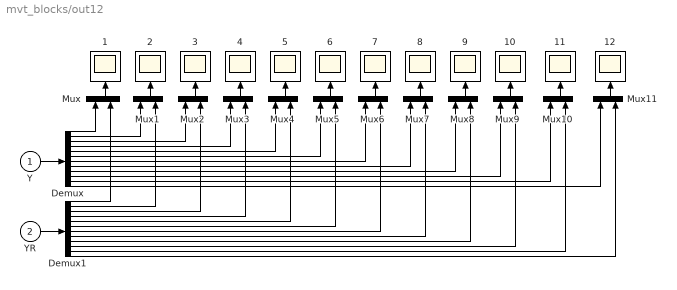
== system mvt_blocks/out12 ==
  Y : Inport  Port=1  PortWidth=-1  SampleTime=0  DataType=auto
      settings: SignalType=auto
  YR : Inport  Port=2  PortWidth=-1  SampleTime=0  DataType=auto
      settings: SignalType=auto
   {1..12} (12 alike) : Scope
      " 1" settings: Orientation=up  TimeRange=100.000000  YMin=-2  YMax=2  SaveToWorkspace=off  SaveName=ScopeData  DataFormat=Matrix
      " 10" settings: Orientation=up  TimeRange=100.000000  YMin=-2.000000  YMax=2.000000  SaveToWorkspace=off  SaveName=ScopeData  DataFormat=Matrix
      " 11" settings: Orientation=up  TimeRange=100.000000  YMin=-2.000000  YMax=2.000000  SaveToWorkspace=off  SaveName=ScopeData  DataFormat=Matrix
      " 12" settings: Orientation=up  TimeRange=100.000000  YMin=-2.000000  YMax=2.000000  SaveToWorkspace=off  SaveName=ScopeData  DataFormat=Matrix
      " 2" settings: Orientation=up  TimeRange=100.000000  YMin=-2.000000  YMax=2.000000  SaveToWorkspace=off  SaveName=ScopeData  DataFormat=Matrix
      " 3" settings: Orientation=up  TimeRange=100.000000  YMin=-2.000000  YMax=2.000000  SaveToWorkspace=off  SaveName=ScopeData  DataFormat=Matrix
      " 4" settings: Orientation=up  TimeRange=100.000000  YMin=-2.000000  YMax=2.000000  SaveToWorkspace=off  SaveName=ScopeData  DataFormat=Matrix
      " 5" settings: Orientation=up  TimeRange=100.000000  YMin=-2.000000  YMax=2.000000  SaveToWorkspace=off  SaveName=ScopeData  DataFormat=Matrix
      " 6" settings: Orientation=up  TimeRange=100.000000  YMin=-2.000000  YMax=2.000000  SaveToWorkspace=off  SaveName=ScopeData  DataFormat=Matrix
      " 7" settings: Orientation=up  TimeRange=100.000000  YMin=-2.000000  YMax=2.000000  SaveToWorkspace=off  SaveName=ScopeData  DataFormat=Matrix
      " 8" settings: Orientation=up  TimeRange=100.000000  YMin=-2.000000  YMax=2.000000  SaveToWorkspace=off  SaveName=ScopeData  DataFormat=Matrix
      " 9" settings: Orientation=up  TimeRange=100.000000  YMin=-2.000000  YMax=2.000000  SaveToWorkspace=off  SaveName=ScopeData  DataFormat=Matrix
  Demux : Demux  Outputs=12
  Demux1 : Demux  Outputs=12
  Mux{,1..11} (12 alike) : Mux  Orientation=up  Inputs=2
  wires:
  Demux1/11 -> Mux10/2
  Demux/11 -> Mux10/1
  Mux10/1 -> " 11"/1
  Demux1/10 -> Mux9/2
  Demux/10 -> Mux9/1
  Mux9/1 -> " 10"/1
  Demux1/4 -> Mux3/2
  Demux1/9 -> Mux8/2
  Demux/9 -> Mux8/1
  Mux8/1 -> " 9"/1
  Demux1/1 -> Mux/2
  Demux1/8 -> Mux7/2
  Demux/8 -> Mux7/1
  Mux7/1 -> " 8"/1
  Mux6/1 -> " 7"/1
  Mux5/1 -> " 6"/1
  Mux4/1 -> " 5"/1
  Mux3/1 -> " 4"/1
  Mux2/1 -> " 3"/1
  Mux1/1 -> " 2"/1
  Demux1/7 -> Mux6/2
  Demux/7 -> Mux6/1
  Demux1/6 -> Mux5/2
  Demux/6 -> Mux5/1
  Demux1/5 -> Mux4/2
  Demux/5 -> Mux4/1
  Demux/2 -> Mux1/1
  Demux/4 -> Mux3/1
  Demux1/3 -> Mux2/2
  Demux1/2 -> Mux1/2
  YR/1 -> Demux1/1
  Demux/1 -> Mux/1
  Demux/3 -> Mux2/1
  Mux/1 -> " 1"/1
  Y/1 -> Demux/1
  Mux11/1 -> " 12"/1
  Demux/12 -> Mux11/1
  Demux1/12 -> Mux11/2

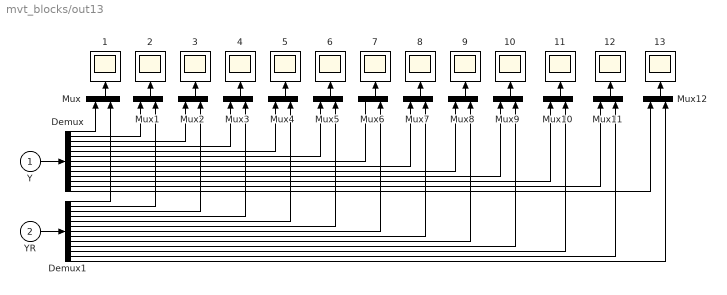
== system mvt_blocks/out13 ==
  Y : Inport  Port=1  PortWidth=-1  SampleTime=0  DataType=auto
      settings: SignalType=auto
  YR : Inport  Port=2  PortWidth=-1  SampleTime=0  DataType=auto
      settings: SignalType=auto
   {1..13} (13 alike) : Scope
      " 1" settings: Orientation=up  TimeRange=100.000000  YMin=-2  YMax=2  SaveToWorkspace=off  SaveName=ScopeData  DataFormat=Matrix
      " 10" settings: Orientation=up  TimeRange=100.000000  YMin=-2.000000  YMax=2.000000  SaveToWorkspace=off  SaveName=ScopeData  DataFormat=Matrix
      " 11" settings: Orientation=up  TimeRange=100.000000  YMin=-2.000000  YMax=2.000000  SaveToWorkspace=off  SaveName=ScopeData  DataFormat=Matrix
      " 12" settings: Orientation=up  TimeRange=100.000000  YMin=-2.000000  YMax=2.000000  SaveToWorkspace=off  SaveName=ScopeData  DataFormat=Matrix
      " 13" settings: Orientation=up  TimeRange=100.000000  YMin=-2.000000  YMax=2.000000  SaveToWorkspace=off  SaveName=ScopeData  DataFormat=Matrix
      " 2" settings: Orientation=up  TimeRange=100.000000  YMin=-2.000000  YMax=2.000000  SaveToWorkspace=off  SaveName=ScopeData  DataFormat=Matrix
      " 3" settings: Orientation=up  TimeRange=100.000000  YMin=-2.000000  YMax=2.000000  SaveToWorkspace=off  SaveName=ScopeData  DataFormat=Matrix
      " 4" settings: Orientation=up  TimeRange=100.000000  YMin=-2.000000  YMax=2.000000  SaveToWorkspace=off  SaveName=ScopeData  DataFormat=Matrix
      " 5" settings: Orientation=up  TimeRange=100.000000  YMin=-2.000000  YMax=2.000000  SaveToWorkspace=off  SaveName=ScopeData  DataFormat=Matrix
      " 6" settings: Orientation=up  TimeRange=100.000000  YMin=-2.000000  YMax=2.000000  SaveToWorkspace=off  SaveName=ScopeData  DataFormat=Matrix
      " 7" settings: Orientation=up  TimeRange=100.000000  YMin=-2.000000  YMax=2.000000  SaveToWorkspace=off  SaveName=ScopeData  DataFormat=Matrix
      " 8" settings: Orientation=up  TimeRange=100.000000  YMin=-2.000000  YMax=2.000000  SaveToWorkspace=off  SaveName=ScopeData  DataFormat=Matrix
      " 9" settings: Orientation=up  TimeRange=100.000000  YMin=-2.000000  YMax=2.000000  SaveToWorkspace=off  SaveName=ScopeData  DataFormat=Matrix
  Demux : Demux  Outputs=13
  Demux1 : Demux  Outputs=13
  Mux{,1..12} (13 alike) : Mux  Orientation=up  Inputs=2
  wires:
  Demux1/12 -> Mux11/2
  Demux/12 -> Mux11/1
  Mux11/1 -> " 12"/1
  Y/1 -> Demux/1
  Mux/1 -> " 1"/1
  Demux/3 -> Mux2/1
  Demux/1 -> Mux/1
  YR/1 -> Demux1/1
  Demux1/2 -> Mux1/2
  Demux1/3 -> Mux2/2
  Demux/4 -> Mux3/1
  Demux/2 -> Mux1/1
  Demux/5 -> Mux4/1
  Demux1/5 -> Mux4/2
  Demux/6 -> Mux5/1
  Demux1/6 -> Mux5/2
  Demux1/7 -> Mux6/2
  Mux1/1 -> " 2"/1
  Mux2/1 -> " 3"/1
  Mux3/1 -> " 4"/1
  Mux4/1 -> " 5"/1
  Mux5/1 -> " 6"/1
  Mux6/1 -> " 7"/1
  Mux7/1 -> " 8"/1
  Demux/8 -> Mux7/1
  Demux1/8 -> Mux7/2
  Demux1/1 -> Mux/2
  Mux8/1 -> " 9"/1
  Demux/9 -> Mux8/1
  Demux1/9 -> Mux8/2
  Demux1/4 -> Mux3/2
  Mux9/1 -> " 10"/1
  Demux/10 -> Mux9/1
  Demux1/10 -> Mux9/2
  Mux10/1 -> " 11"/1
  Demux/11 -> Mux10/1
  Demux1/11 -> Mux10/2
  Mux12/1 -> " 13"/1
  Demux/13 -> Mux12/1
  Demux1/13 -> Mux12/2
  Demux/7 -> ?

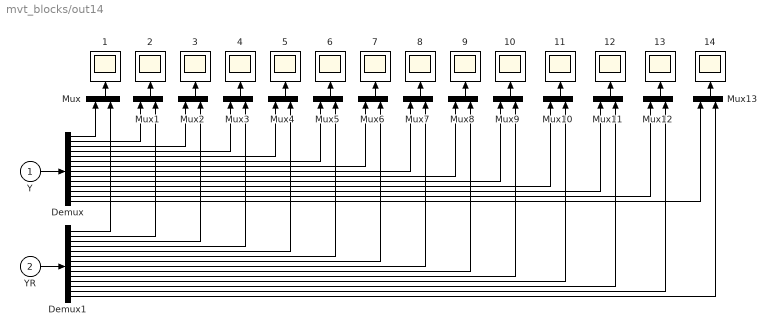
== system mvt_blocks/out14 ==
  Y : Inport  Port=1  PortWidth=-1  SampleTime=0  DataType=auto
      settings: SignalType=auto
  YR : Inport  Port=2  PortWidth=-1  SampleTime=0  DataType=auto
      settings: SignalType=auto
   {1..14} (14 alike) : Scope
      " 1" settings: Orientation=up  TimeRange=100.000000  YMin=-2  YMax=2  SaveToWorkspace=off  SaveName=ScopeData  DataFormat=Matrix
      " 10" settings: Orientation=up  TimeRange=100.000000  YMin=-2.000000  YMax=2.000000  SaveToWorkspace=off  SaveName=ScopeData  DataFormat=Matrix
      " 11" settings: Orientation=up  TimeRange=100.000000  YMin=-2.000000  YMax=2.000000  SaveToWorkspace=off  SaveName=ScopeData  DataFormat=Matrix
      " 12" settings: Orientation=up  TimeRange=100.000000  YMin=-2.000000  YMax=2.000000  SaveToWorkspace=off  SaveName=ScopeData  DataFormat=Matrix
      " 13" settings: Orientation=up  TimeRange=100.000000  YMin=-2.000000  YMax=2.000000  SaveToWorkspace=off  SaveName=ScopeData  DataFormat=Matrix
      " 14" settings: Orientation=up  TimeRange=100.000000  YMin=-2.000000  YMax=2.000000  SaveToWorkspace=off  SaveName=ScopeData  DataFormat=Matrix
      " 2" settings: Orientation=up  TimeRange=100.000000  YMin=-2.000000  YMax=2.000000  SaveToWorkspace=off  SaveName=ScopeData  DataFormat=Matrix
      " 3" settings: Orientation=up  TimeRange=100.000000  YMin=-2.000000  YMax=2.000000  SaveToWorkspace=off  SaveName=ScopeData  DataFormat=Matrix
      " 4" settings: Orientation=up  TimeRange=100.000000  YMin=-2.000000  YMax=2.000000  SaveToWorkspace=off  SaveName=ScopeData  DataFormat=Matrix
      " 5" settings: Orientation=up  TimeRange=100.000000  YMin=-2.000000  YMax=2.000000  SaveToWorkspace=off  SaveName=ScopeData  DataFormat=Matrix
      " 6" settings: Orientation=up  TimeRange=100.000000  YMin=-2.000000  YMax=2.000000  SaveToWorkspace=off  SaveName=ScopeData  DataFormat=Matrix
      " 7" settings: Orientation=up  TimeRange=100.000000  YMin=-2.000000  YMax=2.000000  SaveToWorkspace=off  SaveName=ScopeData  DataFormat=Matrix
      " 8" settings: Orientation=up  TimeRange=100.000000  YMin=-2.000000  YMax=2.000000  SaveToWorkspace=off  SaveName=ScopeData  DataFormat=Matrix
      " 9" settings: Orientation=up  TimeRange=100.000000  YMin=-2.000000  YMax=2.000000  SaveToWorkspace=off  SaveName=ScopeData  DataFormat=Matrix
  Demux : Demux  Outputs=14
  Demux1 : Demux  Outputs=14
  Mux{,1..13} (14 alike) : Mux  Orientation=up  Inputs=2
  wires:
  Demux1/13 -> Mux12/2
  Demux/13 -> Mux12/1
  Mux12/1 -> " 13"/1
  Demux1/11 -> Mux10/2
  Demux/11 -> Mux10/1
  Mux10/1 -> " 11"/1
  Demux1/10 -> Mux9/2
  Demux/10 -> Mux9/1
  Mux9/1 -> " 10"/1
  Demux1/4 -> Mux3/2
  Demux1/9 -> Mux8/2
  Demux/9 -> Mux8/1
  Mux8/1 -> " 9"/1
  Demux1/1 -> Mux/2
  Demux1/8 -> Mux7/2
  Demux/8 -> Mux7/1
  Mux7/1 -> " 8"/1
  Mux6/1 -> " 7"/1
  Mux5/1 -> " 6"/1
  Mux4/1 -> " 5"/1
  Mux3/1 -> " 4"/1
  Mux2/1 -> " 3"/1
  Mux1/1 -> " 2"/1
  Demux1/7 -> Mux6/2
  Demux/7 -> Mux6/1
  Demux1/6 -> Mux5/2
  Demux/6 -> Mux5/1
  Demux1/5 -> Mux4/2
  Demux/5 -> Mux4/1
  Demux/2 -> Mux1/1
  Demux/4 -> Mux3/1
  Demux1/3 -> Mux2/2
  Demux1/2 -> Mux1/2
  YR/1 -> Demux1/1
  Demux/1 -> Mux/1
  Demux/3 -> Mux2/1
  Mux/1 -> " 1"/1
  Y/1 -> Demux/1
  Mux11/1 -> " 12"/1
  Demux/12 -> Mux11/1
  Demux1/12 -> Mux11/2
  Mux13/1 -> " 14"/1
  Demux/14 -> Mux13/1
  Demux1/14 -> Mux13/2

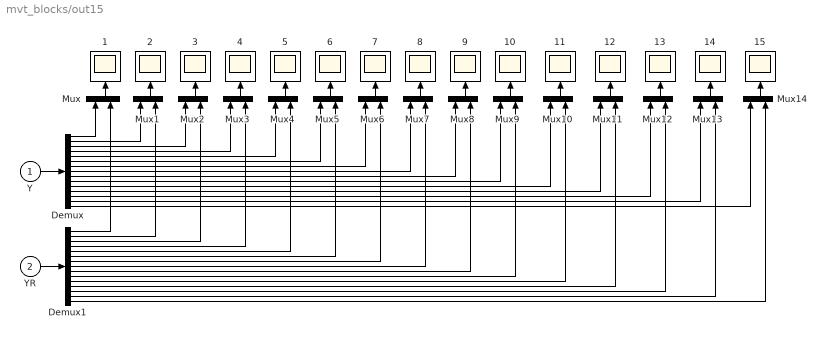
== system mvt_blocks/out15 ==
  Y : Inport  Port=1  PortWidth=-1  SampleTime=0  DataType=auto
      settings: SignalType=auto
  YR : Inport  Port=2  PortWidth=-1  SampleTime=0  DataType=auto
      settings: SignalType=auto
   {1..15} (15 alike) : Scope
      " 1" settings: Orientation=up  TimeRange=100.000000  YMin=-2  YMax=2  SaveToWorkspace=off  SaveName=ScopeData  DataFormat=Matrix
      " 10" settings: Orientation=up  TimeRange=100.000000  YMin=-2.000000  YMax=2.000000  SaveToWorkspace=off  SaveName=ScopeData  DataFormat=Matrix
      " 11" settings: Orientation=up  TimeRange=100.000000  YMin=-2.000000  YMax=2.000000  SaveToWorkspace=off  SaveName=ScopeData  DataFormat=Matrix
      " 12" settings: Orientation=up  TimeRange=100.000000  YMin=-2.000000  YMax=2.000000  SaveToWorkspace=off  SaveName=ScopeData  DataFormat=Matrix
      " 13" settings: Orientation=up  TimeRange=100.000000  YMin=-2.000000  YMax=2.000000  SaveToWorkspace=off  SaveName=ScopeData  DataFormat=Matrix
      " 14" settings: Orientation=up  TimeRange=100.000000  YMin=-2.000000  YMax=2.000000  SaveToWorkspace=off  SaveName=ScopeData  DataFormat=Matrix
      " 15" settings: Orientation=up  TimeRange=100.000000  YMin=-2.000000  YMax=2.000000  SaveToWorkspace=off  SaveName=ScopeData  DataFormat=Matrix
      " 2" settings: Orientation=up  TimeRange=100.000000  YMin=-2.000000  YMax=2.000000  SaveToWorkspace=off  SaveName=ScopeData  DataFormat=Matrix
      " 3" settings: Orientation=up  TimeRange=100.000000  YMin=-2.000000  YMax=2.000000  SaveToWorkspace=off  SaveName=ScopeData  DataFormat=Matrix
      " 4" settings: Orientation=up  TimeRange=100.000000  YMin=-2.000000  YMax=2.000000  SaveToWorkspace=off  SaveName=ScopeData  DataFormat=Matrix
      " 5" settings: Orientation=up  TimeRange=100.000000  YMin=-2.000000  YMax=2.000000  SaveToWorkspace=off  SaveName=ScopeData  DataFormat=Matrix
      " 6" settings: Orientation=up  TimeRange=100.000000  YMin=-2.000000  YMax=2.000000  SaveToWorkspace=off  SaveName=ScopeData  DataFormat=Matrix
      " 7" settings: Orientation=up  TimeRange=100.000000  YMin=-2.000000  YMax=2.000000  SaveToWorkspace=off  SaveName=ScopeData  DataFormat=Matrix
      " 8" settings: Orientation=up  TimeRange=100.000000  YMin=-2.000000  YMax=2.000000  SaveToWorkspace=off  SaveName=ScopeData  DataFormat=Matrix
      " 9" settings: Orientation=up  TimeRange=100.000000  YMin=-2.000000  YMax=2.000000  SaveToWorkspace=off  SaveName=ScopeData  DataFormat=Matrix
  Demux : Demux  Outputs=15
  Demux1 : Demux  Outputs=15
  Mux{,1..14} (15 alike) : Mux  Orientation=up  Inputs=2
  wires:
  Demux1/14 -> Mux13/2
  Demux/14 -> Mux13/1
  Mux13/1 -> " 14"/1
  Demux1/12 -> Mux11/2
  Demux/12 -> Mux11/1
  Mux11/1 -> " 12"/1
  Y/1 -> Demux/1
  Mux/1 -> " 1"/1
  Demux/3 -> Mux2/1
  Demux/1 -> Mux/1
  YR/1 -> Demux1/1
  Demux1/2 -> Mux1/2
  Demux1/3 -> Mux2/2
  Demux/4 -> Mux3/1
  Demux/2 -> Mux1/1
  Demux/5 -> Mux4/1
  Demux1/5 -> Mux4/2
  Demux/6 -> Mux5/1
  Demux1/6 -> Mux5/2
  Demux/7 -> Mux6/1
  Demux1/7 -> Mux6/2
  Mux1/1 -> " 2"/1
  Mux2/1 -> " 3"/1
  Mux3/1 -> " 4"/1
  Mux4/1 -> " 5"/1
  Mux5/1 -> " 6"/1
  Mux6/1 -> " 7"/1
  Mux7/1 -> " 8"/1
  Demux/8 -> Mux7/1
  Demux1/8 -> Mux7/2
  Demux1/1 -> Mux/2
  Mux8/1 -> " 9"/1
  Demux/9 -> Mux8/1
  Demux1/9 -> Mux8/2
  Demux1/4 -> Mux3/2
  Mux9/1 -> " 10"/1
  Demux/10 -> Mux9/1
  Demux1/10 -> Mux9/2
  Mux10/1 -> " 11"/1
  Demux/11 -> Mux10/1
  Demux1/11 -> Mux10/2
  Mux12/1 -> " 13"/1
  Demux/13 -> Mux12/1
  Demux1/13 -> Mux12/2
  Mux14/1 -> " 15"/1
  Demux/15 -> Mux14/1
  Demux1/15 -> Mux14/2

== system mvt_blocks/out2 ==
  Y : Inport  Port=1  PortWidth=-1  SampleTime=0  DataType=auto
      settings: SignalType=auto
  YR : Inport  Port=2  PortWidth=-1  SampleTime=0  DataType=auto
      settings: SignalType=auto
  " 1" : Scope
      settings: Orientation=up  TimeRange=100.000000  YMin=-2  YMax=2  SaveToWorkspace=off  SaveName=ScopeData  DataFormat=Matrix
  " 2" : Scope
      settings: Orientation=up  TimeRange=100.000000  YMin=-2.000000  YMax=2.000000  SaveToWorkspace=off  SaveName=ScopeData  DataFormat=Matrix
  Demux : Demux  Outputs=2
  Demux1 : Demux  Outputs=2
  Mux : Mux  Orientation=up  Inputs=2
  Mux1 : Mux  Orientation=up  Inputs=2
  wires:
  Demux/2 -> Mux1/1
  Demux1/2 -> Mux1/2
  Demux1/1 -> Mux/2
  YR/1 -> Demux1/1
  Demux/1 -> Mux/1
  Mux1/1 -> " 2"/1
  Mux/1 -> " 1"/1
  Y/1 -> Demux/1

== system mvt_blocks/out3 ==
  Y : Inport  Port=1  PortWidth=-1  SampleTime=0  DataType=auto
      settings: SignalType=auto
  YR : Inport  Port=2  PortWidth=-1  SampleTime=0  DataType=auto
      settings: SignalType=auto
  " 1" : Scope
      settings: Orientation=up  TimeRange=100.000000  YMin=-2  YMax=2  SaveToWorkspace=off  SaveName=ScopeData  DataFormat=Matrix
  " 2" : Scope
      settings: Orientation=up  TimeRange=100.000000  YMin=-2.000000  YMax=2.000000  SaveToWorkspace=off  SaveName=ScopeData  DataFormat=Matrix
  " 3" : Scope
      settings: Orientation=up  TimeRange=100.000000  YMin=-2.000000  YMax=2.000000  SaveToWorkspace=off  SaveName=ScopeData  DataFormat=Matrix
  Demux : Demux  Outputs=3
  Demux1 : Demux  Outputs=3
  Mux : Mux  Orientation=up  Inputs=2
  Mux1 : Mux  Orientation=up  Inputs=2
  Mux2 : Mux  Orientation=up  Inputs=2
  wires:
  Y/1 -> Demux/1
  Mux/1 -> " 1"/1
  Mux1/1 -> " 2"/1
  Mux2/1 -> " 3"/1
  Demux/3 -> Mux2/1
  Demux/1 -> Mux/1
  YR/1 -> Demux1/1
  Demux1/1 -> Mux/2
  Demux1/2 -> Mux1/2
  Demux1/3 -> Mux2/2
  Demux/2 -> Mux1/1

== system mvt_blocks/out4 ==
  Y : Inport  Port=1  PortWidth=-1  SampleTime=0  DataType=auto
      settings: SignalType=auto
  YR : Inport  Port=2  PortWidth=-1  SampleTime=0  DataType=auto
      settings: SignalType=auto
   {1..4} (4 alike) : Scope
      " 1" settings: Orientation=up  TimeRange=100.000000  YMin=-2  YMax=2  SaveToWorkspace=off  SaveName=ScopeData  DataFormat=Matrix
      " 2" settings: Orientation=up  TimeRange=100.000000  YMin=-2.000000  YMax=2.000000  SaveToWorkspace=off  SaveName=ScopeData  DataFormat=Matrix
      " 3" settings: Orientation=up  TimeRange=100.000000  YMin=-2.000000  YMax=2.000000  SaveToWorkspace=off  SaveName=ScopeData  DataFormat=Matrix
      " 4" settings: Orientation=up  TimeRange=100.000000  YMin=-2.000000  YMax=2.000000  SaveToWorkspace=off  SaveName=ScopeData  DataFormat=Matrix
  Demux : Demux  Outputs=4
  Demux1 : Demux  Outputs=4
  Mux{,1..3} (4 alike) : Mux  Orientation=up  Inputs=2
  wires:
  Demux/2 -> Mux1/1
  Demux1/4 -> Mux3/2
  Demux/4 -> Mux3/1
  Mux3/1 -> " 4"/1
  Demux1/3 -> Mux2/2
  Demux1/1 -> Mux/2
  YR/1 -> Demux1/1
  Demux/3 -> Mux2/1
  Mux2/1 -> " 3"/1
  Mux1/1 -> " 2"/1
  Mux/1 -> " 1"/1
  Y/1 -> Demux/1
  Demux/1 -> Mux/1
  Demux1/2 -> Mux1/2

== system mvt_blocks/out5 ==
  Y : Inport  Port=1  PortWidth=-1  SampleTime=0  DataType=auto
      settings: SignalType=auto
  YR : Inport  Port=2  PortWidth=-1  SampleTime=0  DataType=auto
      settings: SignalType=auto
   {1..5} (5 alike) : Scope
      " 1" settings: Orientation=up  TimeRange=100.000000  YMin=-2  YMax=2  SaveToWorkspace=off  SaveName=ScopeData  DataFormat=Matrix
      " 2" settings: Orientation=up  TimeRange=100.000000  YMin=-2.000000  YMax=2.000000  SaveToWorkspace=off  SaveName=ScopeData  DataFormat=Matrix
      " 3" settings: Orientation=up  TimeRange=100.000000  YMin=-2.000000  YMax=2.000000  SaveToWorkspace=off  SaveName=ScopeData  DataFormat=Matrix
      " 4" settings: Orientation=up  TimeRange=100.000000  YMin=-2.000000  YMax=2.000000  SaveToWorkspace=off  SaveName=ScopeData  DataFormat=Matrix
      " 5" settings: Orientation=up  TimeRange=100.000000  YMin=-2.000000  YMax=2.000000  SaveToWorkspace=off  SaveName=ScopeData  DataFormat=Matrix
  Demux : Demux  Outputs=5
  Demux1 : Demux  Outputs=5
  Mux{,1..4} (5 alike) : Mux  Orientation=up  Inputs=2
  wires:
  Y/1 -> Demux/1
  Mux/1 -> " 1"/1
  Mux1/1 -> " 2"/1
  Mux2/1 -> " 3"/1
  Demux/3 -> Mux2/1
  Demux/1 -> Mux/1
  YR/1 -> Demux1/1
  Demux1/1 -> Mux/2
  Demux1/3 -> Mux2/2
  Mux3/1 -> " 4"/1
  Demux/4 -> Mux3/1
  Demux1/4 -> Mux3/2
  Demux/2 -> Mux1/1
  Mux4/1 -> " 5"/1
  Demux/5 -> Mux4/1
  Demux1/5 -> Mux4/2
  Demux1/2 -> Mux1/2

== system mvt_blocks/out6 ==
  Y : Inport  Port=1  PortWidth=-1  SampleTime=0  DataType=auto
      settings: SignalType=auto
  YR : Inport  Port=2  PortWidth=-1  SampleTime=0  DataType=auto
      settings: SignalType=auto
   {1..6} (6 alike) : Scope
      " 1" settings: Orientation=up  TimeRange=100.000000  YMin=-2  YMax=2  SaveToWorkspace=off  SaveName=ScopeData  DataFormat=Matrix
      " 2" settings: Orientation=up  TimeRange=100.000000  YMin=-2.000000  YMax=2.000000  SaveToWorkspace=off  SaveName=ScopeData  DataFormat=Matrix
      " 3" settings: Orientation=up  TimeRange=100.000000  YMin=-2.000000  YMax=2.000000  SaveToWorkspace=off  SaveName=ScopeData  DataFormat=Matrix
      " 4" settings: Orientation=up  TimeRange=100.000000  YMin=-2.000000  YMax=2.000000  SaveToWorkspace=off  SaveName=ScopeData  DataFormat=Matrix
      " 5" settings: Orientation=up  TimeRange=100.000000  YMin=-2.000000  YMax=2.000000  SaveToWorkspace=off  SaveName=ScopeData  DataFormat=Matrix
      " 6" settings: Orientation=up  TimeRange=100.000000  YMin=-2.000000  YMax=2.000000  SaveToWorkspace=off  SaveName=ScopeData  DataFormat=Matrix
  Demux : Demux  Outputs=6
  Demux1 : Demux  Outputs=6
  Mux{,1..5} (6 alike) : Mux  Orientation=up  Inputs=2
  wires:
  Y/1 -> Demux/1
  Mux/1 -> " 1"/1
  Mux1/1 -> " 2"/1
  Mux2/1 -> " 3"/1
  Demux/3 -> Mux2/1
  Demux/1 -> Mux/1
  YR/1 -> Demux1/1
  Demux1/1 -> Mux/2
  Demux1/2 -> Mux1/2
  Demux1/3 -> Mux2/2
  Mux3/1 -> " 4"/1
  Demux/4 -> Mux3/1
  Demux1/4 -> Mux3/2
  Demux/2 -> Mux1/1
  Demux/5 -> Mux4/1
  Demux1/5 -> Mux4/2
  Mux4/1 -> " 5"/1
  Mux5/1 -> " 6"/1
  Demux/6 -> Mux5/1
  Demux1/6 -> Mux5/2
